simulink model "RobotFaultDetection_Phase1_step10_baseline_PASS"  (R2026a)
settings: Solver=ode23t  StopTime=20  MaxStep=1e-3  RelTol=1e-4  AbsTol=1e-6
model workspace: external: MAT-File C:\Users\AMMAR\Documents\MATLAB\Digital twin Predictive maintenance\models\Physical\GDOFrobot_DataFile.mat (data not in the file)
undefined symbols (not defined in the file or in its folder): smiData, X, Y, Z
libraries: sm_lib x42, nesl_utility x20, simulink x3
(part 2 of 2)

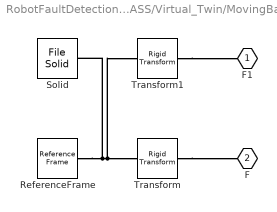
== system RobotFaultDetection_Phase1_step10_baseline_PASS/Virtual_Twin/MovingBase ==
  ReferenceFrame : sm_lib/Frames and Transforms/Reference Frame
  Solid : sm_lib/Body Elements/File Solid  ExtGeomFileName=base_joint_Default_sldprt.STEP  UnitType=FromFile  ExtGeomFileUnits=m  StepReaderType=HEX  ExportConvexHullGeometry=off  InertiaType=Custom  BasedOnType=DensityFromFile  Density=1000  DensityUnits=kg/m^3  Mass=smiData.Solid(1).mass  MassUnits=kg  CenterOfMass=smiData.Solid(1).CoM  CenterOfMassUnits=mm  MomentsOfInertia=smiData.Solid(1).MoI  MomentsOfInertiaUnits=kg*mm^2  ProductsOfInertia=smiData.Solid(1).PoI  ProductsOfInertiaUnits=kg*mm^2  GraphicType=FromGeometry  MarkerShape=Sphere  MarkerSize=10  GraphicVisPropType=SimpleVisualProperties  GraphicDiffuseColor=smiData.Solid(1).color  GraphicOpacity=smiData.Solid(1).opacity  GraphicSpecularColor=[0.5 0.5 0.5 1.0]  GraphicAmbientColor=[0.15 0.15 0.15 1.0]  GraphicEmissiveColor=[0.0 0.0 0.0 1.0]  GraphicShininess=75  DoExposeReferenceFrame=on  SerializedFrames=<Frames/>
  Transform : sm_lib/Frames and Transforms/Rigid Transform  RotationMethod=ArbitraryAxis  FollAlignAxisA=+X  BaseAlignAxisA=+Y  FollAlignAxisB=+Y  BaseAlignAxisB=+Z  RotationStandardAxis=-Y  RotationAngle=smiData.RigidTransform(3).angle  RotationAngleUnits=rad  RotationArbitraryAxis=smiData.RigidTransform(3).axis  RotationSequenceAxes=FollowerAxes  RotationSequence=XYX  RotationSequenceAngles=[0 0 0]  RotationSequenceAnglesUnits=deg  RotationMatrix=[1 0 0;0 1 0;0 0 1]  Quaternion=[1 0 0 0]  TranslationMethod=Cartesian  TranslationCartesianOffset=smiData.RigidTransform(3).translation  TranslationCartesianOffsetUnits=mm  TranslationStandardAxis=+Z  TranslationStandardOffset=0  TranslationStandardOffsetUnits=m  TranslationROffset=0  TranslationROffsetUnits=m  TranslationThetaOffset=0  TranslationThetaOffsetUnits=deg  TranslationZOffset=0  TranslationZOffsetUnits=m
  Transform1 : sm_lib/Frames and Transforms/Rigid Transform  RotationMethod=ArbitraryAxis  FollAlignAxisA=+X  BaseAlignAxisA=+Y  FollAlignAxisB=+Y  BaseAlignAxisB=+Z  RotationStandardAxis=+Y  RotationAngle=smiData.RigidTransform(5).angle  RotationAngleUnits=rad  RotationArbitraryAxis=smiData.RigidTransform(5).axis  RotationSequenceAxes=FollowerAxes  RotationSequence=XYX  RotationSequenceAngles=[0 0 0]  RotationSequenceAnglesUnits=deg  RotationMatrix=[1 0 0;0 1 0;0 0 1]  Quaternion=[1 0 0 0]  TranslationMethod=Cartesian  TranslationCartesianOffset=smiData.RigidTransform(5).translation  TranslationCartesianOffsetUnits=mm  TranslationStandardAxis=+Z  TranslationStandardOffset=0  TranslationStandardOffsetUnits=m  TranslationROffset=0  TranslationROffsetUnits=m  TranslationThetaOffset=0  TranslationThetaOffsetUnits=deg  TranslationZOffset=0  TranslationZOffsetUnits=m
  F1 : PMIOPort  Side=Right
  F : PMIOPort  Port=2  Side=Right
  connections:
  Solid/RConn1 -- ReferenceFrame/RConn1 -- Transform/LConn1 -- Transform1/LConn1
  Transform/RConn1 -- F/RConn1
  Transform1/RConn1 -- F1/RConn1

== matlab function RobotFaultDetection_Phase1_step10_baseline_PASS/Physical_Arm/MATLAB Function3 ==
  data: tau input; current output
function current = torque_to_current(tau)
    Kt  = 0.1;   % Motor torque constant (Nm/A)
    eta = 0.9;   % Gearbox efficiency
    N   = 100;   % Gear ratio
    current = tau ./ (Kt .* eta .* N);
end

== matlab function RobotFaultDetection_Phase1_step10_baseline_PASS/Physical_Arm/MATLAB Function1 ==
  data: tau input; current output
function current = torque_to_current(tau)
    Kt  = 0.1;   % Motor torque constant (Nm/A)
    eta = 0.9;   % Gearbox efficiency
    N   = 100;   % Gear ratio
    current = tau ./ (Kt .* eta .* N);
end

== matlab function RobotFaultDetection_Phase1_step10_baseline_PASS/Physical_Arm/MATLAB Function2 ==
  data: tau input; current output
function current = torque_to_current(tau)
    Kt  = 0.1;   % Motor torque constant (Nm/A)
    eta = 0.9;   % Gearbox efficiency
    N   = 100;   % Gear ratio
    current = tau ./ (Kt .* eta .* N);
end

== matlab function RobotFaultDetection_Phase1_step10_baseline_PASS/Physical_Arm/PD_Controller/MATLAB Function ==
  data: q_ref input double size=[3 1]; tau output double size=[3 1]; dq_ref input double size=[3 1]; q input double size=[3 1]; dq input double size=[3 1]
function tau = pd_controller(q_ref, dq_ref, q, dq)
%#codegen
% PD + gravity compensation (guide Section 06).
% τ_gravity is a PLACEHOLDER in Phase 0 — replaced by Simscape
% inverse dynamics in Phase 1.

    % ---- Gains (update these after each tuning iteration) ----
    Kp      = [147.42;  153.11;  65];    % [Waist; Shoulder; Elbow]
    Kd      = [ 13.760;   14.291; 6];    % [Waist; Shoulder; Elbow]
    tau_sat = [ 50.0;   50.0;  40.0];    % per-joint torque limits (Nm)

    % ---- Force column vectors (defensive) ----
    q_ref  = q_ref(:);
    dq_ref = dq_ref(:);
    q      = q(:);
    dq     = dq(:);

    % ---- PD control law ----
    e  = q_ref  - q;
    de = dq_ref - dq;

    % --- τ_gravity (Phase 0 placeholder) ---
    tau_g = zeros(3,1);
    tau_g(1) = 0;
    tau_g(2) = -(11.19 * cos(q(2)) + 2.79 * cos(q(2)+q(3)));
    tau_g(3) = -1.9 * ( 2.79 * cos(q(2)+q(3)) );

    tau = Kp .* e + Kd .* de + tau_g;

    % ---- Per-joint torque saturation ----
    tau = max(min(tau, tau_sat), -tau_sat);
end
